simulink model "Propulsion"  (R2024b)
settings: Solver=VariableStepAuto  StartTime=0.0  StopTime=10.0  RelTol=1e-3
values from neighbouring files (symbols this model uses):
  alfa_deg = -1.8    [initACFT_high.m]    (also in init_Cessna.m = 1)
  nrho = 0.75    [initACFT_high.m]    (also in initACFT_low.m; init_Cessna.m)
  nv = 0    [initACFT_high.m]    (also in initACFT_low.m; init_Cessna.m = -1)
  rho_reference_kgpm3 = 1.225    [initACFT_high.m]    (also in init_Cessna.m)
  V_reference_mps = 200    [initACFT_high.m]    (also in init_Cessna.m = 51.4)
  xf_m = -3.8    [initACFT_high.m]    (also in initACFT_low.m; init_Cessna.m = 1)
  zf_m = -0.6    [initACFT_high.m]    (also in initACFT_low.m; init_Cessna.m = 0)
undefined symbols (not defined in the file or in its folder): TMax

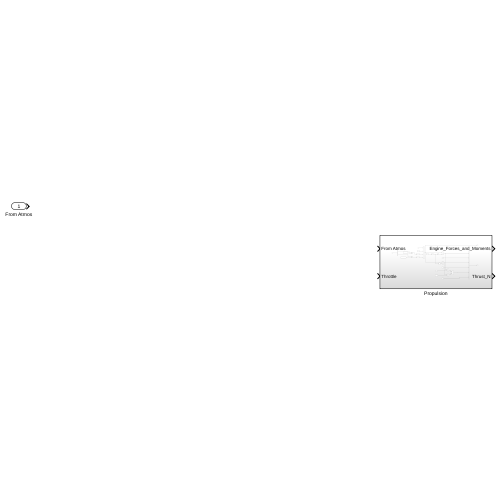
[thumbnail: Simulink's stored preview of the top-level diagram]
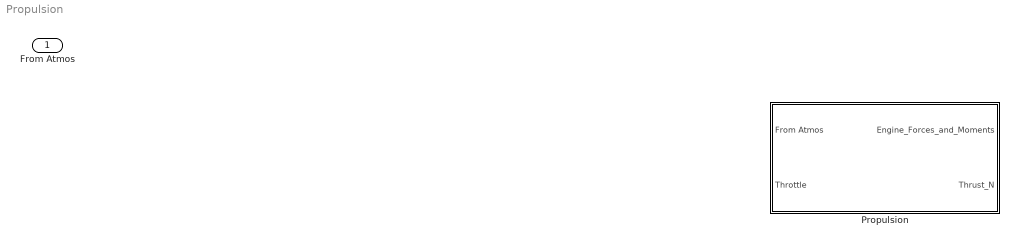
== system Propulsion ==
  From Atmos : Inport
  Propulsion : Subsystem

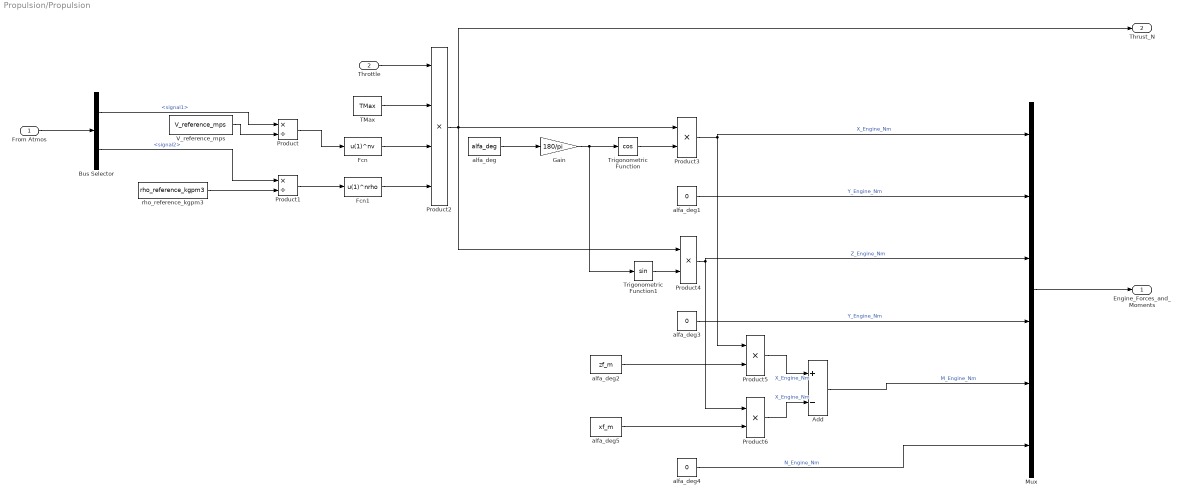
== system Propulsion/Propulsion ==
  From Atmos : Inport
  Throttle : Inport  Port=2
  Add : Sum  Inputs=+-
  Bus Selector : BusSelector  OutputSignals=signal1,signal2
  Fcn : Fcn  Expr=u(1)^nv
  Fcn1 : Fcn  Expr=u(1)^nrho
  Gain : Gain  Gain=180/pi
  Mux : Mux  Inputs=6
  Product : Product  Inputs=*/
  Product1 : Product  Inputs=*/
  Product2 : Product  Inputs=****
  Product{3..6} (4 alike) : Product
  TMax : Constant  Value=TMax
  Trigonometric Function : Trigonometry  Operator=cos
  Trigonometric Function1 : Trigonometry
  V_reference_mps : Constant  Value=V_reference_mps
  alfa_deg : Constant  Value=alfa_deg
  alfa_deg1 : Constant  Value=0
  alfa_deg2 : Constant  Value=zf_m
  alfa_deg3 : Constant  Value=0
  alfa_deg4 : Constant  Value=0
  alfa_deg5 : Constant  Value=xf_m
  rho_reference_kgpm3 : Constant  Value=rho_reference_kgpm3
  Engine_Forces_and_Moments : Outport
  Thrust_N : Outport  Port=2
  wires:
  Throttle/1 -> Product2/1
  Trigonometric Function/1 -> Product3/2
  alfa_deg5/1 -> Product6/2
  alfa_deg2/1 -> Product5/2
  V_reference_mps/1 -> Product/2
  Mux/1 -> Engine_Forces_and_Moments/1
  Product5/1 -> Add/1  "X_Engine_Nm"
  Product6/1 -> Add/2  "X_Engine_Nm"
  rho_reference_kgpm3/1 -> Product1/2
  Product2/1 -> Thrust_N/1, Product4/1, Product3/1
  Product/1 -> Fcn/1
  Product4/1 -> Product6/1, Mux/3  "Z_Engine_Nm"
  From Atmos/1 -> Bus Selector/1
  Product1/1 -> Fcn1/1
  Bus Selector/1 -> Product/1  "<signal1>"
  Gain/1 -> Trigonometric Function1/1, Trigonometric Function/1
  Bus Selector/2 -> Product1/1  "<signal2>"
  alfa_deg4/1 -> Mux/6  "N_Engine_Nm"
  Add/1 -> Mux/5  "M_Engine_Nm"
  Fcn1/1 -> Product2/4
  Trigonometric Function1/1 -> Product4/2
  alfa_deg3/1 -> Mux/4  "Y_Engine_Nm"
  TMax/1 -> Product2/2
  Product3/1 -> Product5/1, Mux/1  "X_Engine_Nm"
  Fcn/1 -> Product2/3
  alfa_deg1/1 -> Mux/2  "Y_Engine_Nm"
  alfa_deg/1 -> Gain/1
